simulink model "STM32_FIR_wrap_sym"  (R2018a)
settings: Solver=FixedStepAuto  StartTime=0.0  StopTime=inf  RelTol=1e-3  EnableMultiTasking=on
libraries: stm32f769ilib x2, mbedblockslib x1
settings Model: SimulationMode=external  Creator=hpong  LastModifiedBy=hpong
settings OptimizationCC: EnhancedBackFolding=on  PassReuseOutputArgsAs=Individual arguments  MaxStackSize=64  OptimizeBlockOrder=speed  DifferentSizesBufferReuse=on  OptimizationCustomize=off
settings DebuggingCC: ParameterTunabilityLossMsg=error
settings HardwareCC: ProdBitPerPointer=32  ProdBitPerSizeT=32  ProdBitPerPtrDiffT=32  ProdLargestAtomicInteger=Long  ProdLargestAtomicFloat=Double  ProdWordSize=32  ProdHWDeviceType=ARM Compatible->ARM Cortex
settings SFSimCC: MATLABDynamicMemAlloc=off
settings RTWCC: SystemTargetFile=ert.tlc  HardwareBoard=STM32F769I-Discovery  TLCOptions=-aInlineSetEventsForThisBaseRateFcn=TLC_FALSE -aSuppressMultiTaskScheduler=TLC_FALSE -aRateBasedStepFcn=1  TemplateMakefile=ert_default_tmf  GenerateReport=on  Toolchain=GNU Tools for ARM Embedded Processors  IncludeHyperlinkInReport=on  LaunchReport=on  GenerateTraceInfo=on  GenerateTraceReport=on  GenerateTraceReportSl=on  GenerateTraceReportSf=on  GenerateTraceReportEml=on
settings CodeAppCC: ForceParamTrailComments=on  IgnoreCustomStorageClasses=off  OperatorAnnotations=on  SimulinkDataObjDesc=on  SFDataObjDesc=on  InsertBlockDesc=on
settings ERTTargetCC: CodeReplacementLibrary=ARM Cortex-M (CMSIS)  SupportComplex=off

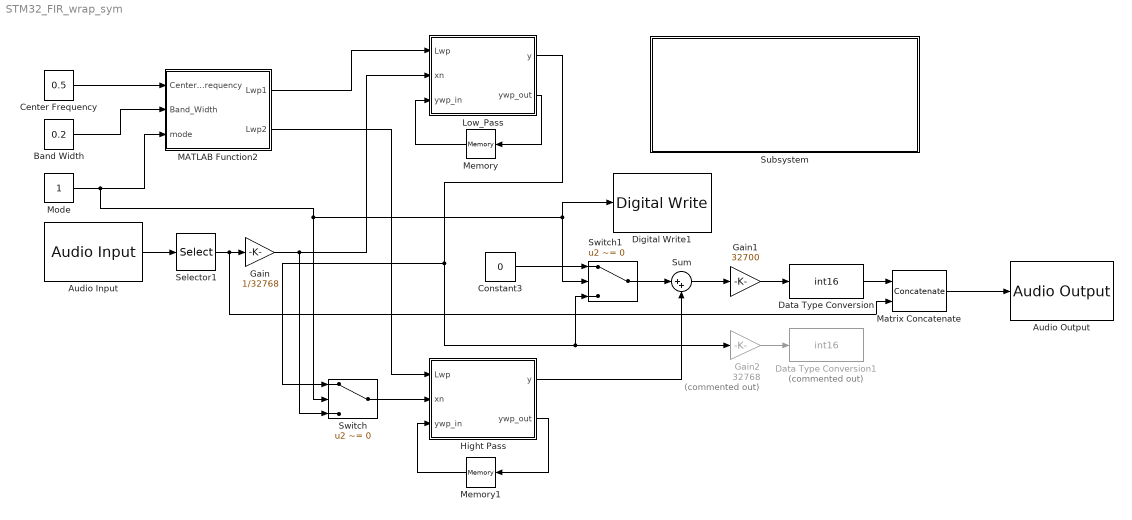
== system STM32_FIR_wrap_sym ==
  Audio Input : stm32f769ilib/Audio Input  InputDevice=LineIn  SamplingFreq=16000  NumCh=2  FrameSize=12
      settings: SourceProductName=Embedded Coder Support Package for STMicroelectronics Discovery Boards  SourceProductBaseCode=STMICRODIS
  Audio Output : stm32f769ilib/Audio Output  OutputDevice=Headphone  SamplingFreq=16000  Volume=64
      settings: SourceProductName=Embedded Coder Support Package for STMicroelectronics Discovery Boards  SourceProductBaseCode=STMICRODIS
  Band Width : Constant  Value=0.2
  Center Frequency : Constant  Value=0.5
  Constant3 : Constant  Value=0
  Data Type Conversion : DataTypeConversion  OutDataTypeStr=int16
  Data Type Conversion1 : DataTypeConversion  Commented=on  OutDataTypeStr=int16
  Digital Write1 : mbedblockslib/Digital Write  Pin=PJ_13  Direction=output
      settings: SourceProductName=Simulink Coder Support Package for BBC microbit Board  SourceProductBaseCode=MICROBIT
  Gain : Gain  Gain=1/32768  OutDataTypeStr=double
  Gain1 : Gain  Gain=32700
  Gain2 : Gain  Commented=on  Gain=32768
  Hight Pass : MATLAB Function  TreatAsAtomicUnit=on
  Low_Pass : MATLAB Function  TreatAsAtomicUnit=on
  MATLAB Function2 : MATLAB Function  TreatAsAtomicUnit=on
  Matrix Concatenate : Concatenate  Mode=Multidimensional array  ConcatenateDimension=2
  Memory : Memory  InitialCondition=[ 0 0 ; 0 0 ; 0 0 ; 0 0 ; 0 0 ; 0 0 ; 0 0 ; 0 0 ; 0 0 ; 0 0 ; 0 0 ; 0 0 ; 0 0 ; 0 0 ; 0 0 ; 0 0 ; 0 0 ; 0 0 ; 0 0 ; 0 0 ; 0 0 ; 0 0 ; 0 0 ; 0 0 ; 0 0 ; 0 0 ; 0 0 ; 0 0 ; 0 0 ; 0 0 ; 0 0 ; 0 0 ; 0 0 ; 0 0 ; 0 0 ; 0 0 ; 0 0 ; 0 0 ; 0 0 ; 0 0 ; 0 0 ; 0 0 ; 0 0 ; 0 0 ; 0 0 ; 0 0 ; 0 0 ; 0 0 ; 0 0 ; 0 0 ; 0 0 ;]  InheritSampleTime=on
  Memory1 : Memory  InitialCondition=[ 0 0 ; 0 0 ; 0 0 ; 0 0 ; 0 0 ; 0 0 ; 0 0 ; 0 0 ; 0 0 ; 0 0 ; 0 0 ; 0 0 ; 0 0 ; 0 0 ; 0 0 ; 0 0 ; 0 0 ; 0 0 ; 0 0 ; 0 0 ; 0 0 ; 0 0 ; 0 0 ; 0 0 ; 0 0 ; 0 0 ; 0 0 ; 0 0 ; 0 0 ; 0 0 ; 0 0 ; 0 0 ; 0 0 ; 0 0 ; 0 0 ; 0 0 ; 0 0 ; 0 0 ; 0 0 ; 0 0 ; 0 0 ; 0 0 ; 0 0 ; 0 0 ; 0 0 ; 0 0 ; 0 0 ; 0 0 ; 0 0 ; 0 0 ; 0 0 ;]  InheritSampleTime=on
  Mode : Constant
  Selector1 : Selector  NumberOfDimensions=2  InputPortWidth=2  IndexOptions=Select all,Index vector (dialog)  Indices=1,1  OutputSizes=1,1
  Subsystem : Subsystem
  Sum : Sum  Inputs=|++
  Switch : Switch  Criteria=u2 ~= 0  Threshold=1
  Switch1 : Switch  Criteria=u2 ~= 0
  wires:
  Matrix Concatenate/1 -> Audio Output/1
  Audio Input/1 -> Selector1/1
  Selector1/1 -> Matrix Concatenate/2, Gain/1
  Gain1/1 -> Data Type Conversion/1
  Data Type Conversion/1 -> Matrix Concatenate/1
  Low_Pass/2(ywp_out) -> Memory/1
  Memory/1 -> Low_Pass/3(ywp_in)
  Memory1/1 -> Hight Pass/3(ywp_in)
  Hight Pass/2(ywp_out) -> Memory1/1
  Gain2/1 -> Data Type Conversion1/1
  Low_Pass/1(y) -> Switch1/3, Gain2/1, Switch/1
  Center Frequency/1 -> MATLAB Function2/1(Center_Frequency)
  Band Width/1 -> MATLAB Function2/2(Band_Width)
  Mode/1 -> Switch1/2, Digital Write1/1, Switch/2, MATLAB Function2/3(mode)
  MATLAB Function2/1(Lwp1) -> Low_Pass/1(Lwp)
  MATLAB Function2/2(Lwp2) -> Hight Pass/1(Lwp)
  Gain/1 -> Switch/3, Low_Pass/2(xn)
  Switch/1 -> Hight Pass/2(xn)
  Sum/1 -> Gain1/1
  Hight Pass/1(y) -> Sum/2
  Switch1/1 -> Sum/1
  Constant3/1 -> Switch1/1

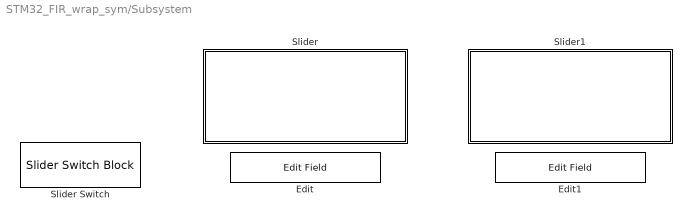
== system STM32_FIR_wrap_sym/Subsystem ==
  Edit : EditField  WebBlockId=137  LabelPosition=Hide  Alignment=Center
  Edit1 : EditField  WebBlockId=138  LabelPosition=Hide  Alignment=Center
  Slider : Subsystem  DialogController=hmiCreateDDGDialog  IsWebBlock=on  mask(MWDashboardBlock){webBlockId=5be6c282-b98e-4823-8651-c7b480b903fc, webBlockType=slider, ShowInLibBrowser=on, ShowInitialText=on, HMISrcModelName=STM32_FIR_wrap_sym}
      mask prompts: webBlockId "WebBlock Id"; webBlockType "WebBlock Type"; HMISrcModelName "Source Model"
      mask help: SimulinkHMI:dialogs:SliderDialogDesc
      mask Help: helpview([docroot '/mapfiles/simulink.map'], 'hmi_slider')
      mask Display:
      | if strcmp(get_param(bdroot(gcb),'BlockDiagramType'), 'library')
      |     image([(matlabroot) '/toolbox/simulink/hmi/icons/Slider.png']);
      | end
  Slider Switch : SliderSwitchBlock  WebBlockId=135
      settings: Values={{'BS', 'BP'}, [0 1]}
  Slider1 : Subsystem  DialogController=hmiCreateDDGDialog  IsWebBlock=on  mask(MWDashboardBlock){webBlockId=f1fd2279-2155-4f04-b89e-48087fd9ee74, webBlockType=slider, ShowInLibBrowser=on, ShowInitialText=on, HMISrcModelName=STM32_FIR_wrap_sym}
      mask prompts: webBlockId "WebBlock Id"; webBlockType "WebBlock Type"; HMISrcModelName "Source Model"
      mask help: SimulinkHMI:dialogs:SliderDialogDesc
      mask Help: helpview([docroot '/mapfiles/simulink.map'], 'hmi_slider')
      mask Display:
      | if strcmp(get_param(bdroot(gcb),'BlockDiagramType'), 'library')
      |     image([(matlabroot) '/toolbox/simulink/hmi/icons/Slider.png']);
      | end

== system STM32_FIR_wrap_sym/Subsystem/Slider ==

== system STM32_FIR_wrap_sym/Subsystem/Slider1 ==

== matlab function STM32_FIR_wrap_sym/Hight Pass ==
  data: Lwp input; xn input; y output; ywp_in input; ywp_out output
function [y, ywp_out] = fir_wrap_high(Lwp,xn, ywp_in)
b = [-0.00101759  -0.00000000  0.00130589  -0.00000000  -0.00207303  -0.00000000  0.00342558  -0.00000000  -0.00549051  -0.00000000  0.00843441  -0.00000000  -0.01250260  -0.00000000  0.01810261  -0.00000000  -0.02600015  -0.00000000  0.03785150  -0.00000000  -0.05801218  -0.00000000  0.10257517  -0.00000000  -0.31684426  0.49950965  -0.31684426  -0.00000000  0.10257517  -0.00000000  -0.05801218  -0.00000000  0.03785150  -0.00000000  -0.02600015  -0.00000000  0.01810261  -0.00000000  -0.01250260  -0.00000000  0.00843441  -0.00000000  -0.00549051  -0.00000000  0.00342558  -0.00000000  -0.00207303  -0.00000000  0.00130589  -0.00000000  -0.00101759  ];
nb = length(b);
half_nb = (nb-1)/2;
y=ones(12,1,'double');
ywp = ywp_in;
xm = [ywp_in(nb,1) ;xn];
for n=2:13
    ywp(1,2) = ywp(1,1);
    ywp(1,1) = (ywp(1,2)-xm(n))*Lwp + xm(n-1);
    for nn=2:nb-1
        ywp(nn,2) = ywp(nn,1);
        ywp(nn,1) = (ywp(nn,2)-ywp(nn-1,1))*Lwp + ywp(nn-1,2);
    end   
    y(n-1)=b(1)*(xm(n)+ ywp(nb-1,1)) + b(half_nb+1)*ywp(half_nb,1);
    for nn=1:half_nb-1
        y(n-1) = y(n-1) + b(nn+1)*(ywp(nn,1) + ywp(nb-1-nn,1) );
    end
end
ywp_out = ywp;
ywp_out(nb,1) = xm(13);
end

== matlab function STM32_FIR_wrap_sym/Low_Pass ==
  data: Lwp input; xn input; y output; ywp_in input; ywp_out output
function [y, ywp_out] = fir_wrap_low(Lwp,xn, ywp_in)
b = [0.00101759  -0.00000000  -0.00130589  0.00000000  0.00207303  -0.00000000  -0.00342558  0.00000000  0.00549051  -0.00000000  -0.00843441  0.00000000  0.01250260  -0.00000000  -0.01810261  0.00000000  0.02600015  -0.00000000  -0.03785150  0.00000000  0.05801218  -0.00000000  -0.10257517  0.00000000  0.31684426  0.49950965  0.31684426  0.00000000  -0.10257517  -0.00000000  0.05801218  0.00000000  -0.03785150  -0.00000000  0.02600015  0.00000000  -0.01810261  -0.00000000  0.01250260  0.00000000  -0.00843441  -0.00000000  0.00549051  0.00000000  -0.00342558  -0.00000000  0.00207303  0.00000000  -0.00130589  -0.00000000  0.00101759  ];
nb = length(b);
half_nb = (nb-1)/2;
y=ones(12,1,'double');
ywp = ywp_in;
xm = [ywp_in(nb,1) ;xn];
for n=2:13
    ywp(1,2) = ywp(1,1);
    ywp(1,1) = (ywp(1,2)-xm(n))*Lwp + xm(n-1);
    for nn=2:nb-1
        ywp(nn,2) = ywp(nn,1);
        ywp(nn,1) = (ywp(nn,2)-ywp(nn-1,1))*Lwp + ywp(nn-1,2);
    end   
    y(n-1)=b(1)*(xm(n)+ ywp(nb-1,1)) + b(half_nb+1)*ywp(half_nb,1);
    for nn=1:half_nb-1
        y(n-1) = y(n-1) + b(nn+1)*(ywp(nn,1) + ywp(nb-1-nn,1) );
    end
end
ywp_out = ywp;
ywp_out(nb,1) = xm(13);
end

== matlab function STM32_FIR_wrap_sym/MATLAB Function2 ==
  data: Center_Frequency input; Band_Width input; Lwp1 output; mode input; Lwp2 output
function [Lwp1, Lwp2] = Lwp_cal(Center_Frequency,Band_Width, mode)
fc1 = 0;
fc2 = 0;
if mode == 0 % Stop Band
    fc1 = Center_Frequency - Band_Width/2 ;%LP
    fc2 = Center_Frequency + Band_Width/2 ;%HP
elseif mode == 1 % Band Pass
    fc1 = Center_Frequency + Band_Width/2 ;%LP
    fc2 = Center_Frequency - Band_Width/2 ;%HP
end
Lwp1 = sin((0.5-fc1).*pi/2)./sin((0.5+fc1).*pi/2);
Lwp2 = sin((0.5-fc2).*pi/2)./sin((0.5+fc2).*pi/2);
end
